simulink model "roach2_5gadc_spec"  (R2013b)
(part 3 of 18)

  pol1_in3_tap3/3(coeff_out) -> pol1_in3_tap4/3(coeff)
  pol1_in3_tap3/4(taps_out) -> adder_1_3/4(din3)
  pol1_in3_tap4/1(dout) -> pol1_in3_tap5/1(din)
  pol1_in3_tap4/2(sync_out) -> pol1_in3_tap5/2(sync)
  pol1_in3_tap4/3(coeff_out) -> pol1_in3_tap5/3(coeff)
  pol1_in3_tap4/4(taps_out) -> adder_1_3/5(din4)
  pol1_in3_tap5/1(dout) -> pol1_in3_tap6/1(din)
  pol1_in3_tap5/2(sync_out) -> pol1_in3_tap6/2(sync)
  pol1_in3_tap5/3(coeff_out) -> pol1_in3_tap6/3(coeff)
  pol1_in3_tap5/4(taps_out) -> adder_1_3/6(din5)
  pol1_in3_tap6/1(dout) -> pol1_in3_tap7/1(din)
  pol1_in3_tap6/2(sync_out) -> pol1_in3_tap7/2(sync)
  pol1_in3_tap6/3(coeff_out) -> pol1_in3_tap7/3(coeff)
  pol1_in3_tap6/4(taps_out) -> adder_1_3/7(din6)
  pol1_in3_last_tap/2(sync_out) -> adder_1_3/1(sync)
  pol1_in3_last_tap/1(tap_out) -> adder_1_3/9(din8)
  pol1_in3_tap7/1(dout) -> pol1_in3_last_tap/1(din)
  pol1_in3_tap7/2(sync_out) -> pol1_in3_last_tap/2(sync)
  pol1_in3_tap7/3(coeff_out) -> pol1_in3_last_tap/3(coeff)
  pol1_in3_tap7/4(taps_out) -> adder_1_3/8(din7)
  pol1_in4_first_tap/1(dout) -> pol1_in4_tap2/1(din)
  pol1_in4_first_tap/2(sync_out) -> pol1_in4_tap2/2(sync)
  pol1_in4_first_tap/3(coeff_out) -> pol1_in4_tap2/3(coeff)
  pol1_in4_first_tap/4(taps_out) -> adder_1_4/2(din1)
  pol1_in4_tap2/1(dout) -> pol1_in4_tap3/1(din)
  pol1_in4_tap2/2(sync_out) -> pol1_in4_tap3/2(sync)
  pol1_in4_tap2/3(coeff_out) -> pol1_in4_tap3/3(coeff)
  pol1_in4_tap2/4(taps_out) -> adder_1_4/3(din2)
  pol1_in4_tap3/1(dout) -> pol1_in4_tap4/1(din)
  pol1_in4_tap3/2(sync_out) -> pol1_in4_tap4/2(sync)
  pol1_in4_tap3/3(coeff_out) -> pol1_in4_tap4/3(coeff)
  pol1_in4_tap3/4(taps_out) -> adder_1_4/4(din3)
  pol1_in4_tap4/1(dout) -> pol1_in4_tap5/1(din)
  pol1_in4_tap4/2(sync_out) -> pol1_in4_tap5/2(sync)
  pol1_in4_tap4/3(coeff_out) -> pol1_in4_tap5/3(coeff)
  pol1_in4_tap4/4(taps_out) -> adder_1_4/5(din4)
  pol1_in4_tap5/1(dout) -> pol1_in4_tap6/1(din)
  pol1_in4_tap5/2(sync_out) -> pol1_in4_tap6/2(sync)
  pol1_in4_tap5/3(coeff_out) -> pol1_in4_tap6/3(coeff)
  pol1_in4_tap5/4(taps_out) -> adder_1_4/6(din5)
  pol1_in4_tap6/1(dout) -> pol1_in4_tap7/1(din)
  pol1_in4_tap6/2(sync_out) -> pol1_in4_tap7/2(sync)
  pol1_in4_tap6/3(coeff_out) -> pol1_in4_tap7/3(coeff)
  pol1_in4_tap6/4(taps_out) -> adder_1_4/7(din6)
  pol1_in4_last_tap/2(sync_out) -> adder_1_4/1(sync)
  pol1_in4_last_tap/1(tap_out) -> adder_1_4/9(din8)
  pol1_in4_tap7/1(dout) -> pol1_in4_last_tap/1(din)
  pol1_in4_tap7/2(sync_out) -> pol1_in4_last_tap/2(sync)
  pol1_in4_tap7/3(coeff_out) -> pol1_in4_last_tap/3(coeff)
  pol1_in4_tap7/4(taps_out) -> adder_1_4/8(din7)
  pol1_in5_first_tap/1(dout) -> pol1_in5_tap2/1(din)
  pol1_in5_first_tap/2(sync_out) -> pol1_in5_tap2/2(sync)
  pol1_in5_first_tap/3(coeff_out) -> pol1_in5_tap2/3(coeff)
  pol1_in5_first_tap/4(taps_out) -> adder_1_5/2(din1)
  pol1_in5_tap2/1(dout) -> pol1_in5_tap3/1(din)
  pol1_in5_tap2/2(sync_out) -> pol1_in5_tap3/2(sync)
  pol1_in5_tap2/3(coeff_out) -> pol1_in5_tap3/3(coeff)
  pol1_in5_tap2/4(taps_out) -> adder_1_5/3(din2)
  pol1_in5_tap3/1(dout) -> pol1_in5_tap4/1(din)
  pol1_in5_tap3/2(sync_out) -> pol1_in5_tap4/2(sync)
  pol1_in5_tap3/3(coeff_out) -> pol1_in5_tap4/3(coeff)
  pol1_in5_tap3/4(taps_out) -> adder_1_5/4(din3)
  pol1_in5_tap4/1(dout) -> pol1_in5_tap5/1(din)
  pol1_in5_tap4/2(sync_out) -> pol1_in5_tap5/2(sync)
  pol1_in5_tap4/3(coeff_out) -> pol1_in5_tap5/3(coeff)
  pol1_in5_tap4/4(taps_out) -> adder_1_5/5(din4)
  pol1_in5_tap5/1(dout) -> pol1_in5_tap6/1(din)
  pol1_in5_tap5/2(sync_out) -> pol1_in5_tap6/2(sync)
  pol1_in5_tap5/3(coeff_out) -> pol1_in5_tap6/3(coeff)
  pol1_in5_tap5/4(taps_out) -> adder_1_5/6(din5)
  pol1_in5_tap6/1(dout) -> pol1_in5_tap7/1(din)
  pol1_in5_tap6/2(sync_out) -> pol1_in5_tap7/2(sync)
  pol1_in5_tap6/3(coeff_out) -> pol1_in5_tap7/3(coeff)
  pol1_in5_tap6/4(taps_out) -> adder_1_5/7(din6)
  pol1_in5_last_tap/2(sync_out) -> adder_1_5/1(sync)
  pol1_in5_last_tap/1(tap_out) -> adder_1_5/9(din8)
  pol1_in5_tap7/1(dout) -> pol1_in5_last_tap/1(din)
  pol1_in5_tap7/2(sync_out) -> pol1_in5_last_tap/2(sync)
  pol1_in5_tap7/3(coeff_out) -> pol1_in5_last_tap/3(coeff)
  pol1_in5_tap7/4(taps_out) -> adder_1_5/8(din7)
  pol1_in6_first_tap/1(dout) -> pol1_in6_tap2/1(din)
  pol1_in6_first_tap/2(sync_out) -> pol1_in6_tap2/2(sync)
  pol1_in6_first_tap/3(coeff_out) -> pol1_in6_tap2/3(coeff)
  pol1_in6_first_tap/4(taps_out) -> adder_1_6/2(din1)
  pol1_in6_tap2/1(dout) -> pol1_in6_tap3/1(din)
  pol1_in6_tap2/2(sync_out) -> pol1_in6_tap3/2(sync)
  pol1_in6_tap2/3(coeff_out) -> pol1_in6_tap3/3(coeff)
  pol1_in6_tap2/4(taps_out) -> adder_1_6/3(din2)
  pol1_in6_tap3/1(dout) -> pol1_in6_tap4/1(din)
  pol1_in6_tap3/2(sync_out) -> pol1_in6_tap4/2(sync)
  pol1_in6_tap3/3(coeff_out) -> pol1_in6_tap4/3(coeff)
  pol1_in6_tap3/4(taps_out) -> adder_1_6/4(din3)
  pol1_in6_tap4/1(dout) -> pol1_in6_tap5/1(din)
  pol1_in6_tap4/2(sync_out) -> pol1_in6_tap5/2(sync)
  pol1_in6_tap4/3(coeff_out) -> pol1_in6_tap5/3(coeff)
  pol1_in6_tap4/4(taps_out) -> adder_1_6/5(din4)
  pol1_in6_tap5/1(dout) -> pol1_in6_tap6/1(din)
  pol1_in6_tap5/2(sync_out) -> pol1_in6_tap6/2(sync)
  pol1_in6_tap5/3(coeff_out) -> pol1_in6_tap6/3(coeff)
  pol1_in6_tap5/4(taps_out) -> adder_1_6/6(din5)
  pol1_in6_tap6/1(dout) -> pol1_in6_tap7/1(din)
  pol1_in6_tap6/2(sync_out) -> pol1_in6_tap7/2(sync)
  pol1_in6_tap6/3(coeff_out) -> pol1_in6_tap7/3(coeff)
  pol1_in6_tap6/4(taps_out) -> adder_1_6/7(din6)
  pol1_in6_last_tap/2(sync_out) -> adder_1_6/1(sync)
  pol1_in6_last_tap/1(tap_out) -> adder_1_6/9(din8)
  pol1_in6_tap7/1(dout) -> pol1_in6_last_tap/1(din)
  pol1_in6_tap7/2(sync_out) -> pol1_in6_last_tap/2(sync)
  pol1_in6_tap7/3(coeff_out) -> pol1_in6_last_tap/3(coeff)
  pol1_in6_tap7/4(taps_out) -> adder_1_6/8(din7)
  pol1_in7_first_tap/1(dout) -> pol1_in7_tap2/1(din)
  pol1_in7_first_tap/2(sync_out) -> pol1_in7_tap2/2(sync)
  pol1_in7_first_tap/3(coeff_out) -> pol1_in7_tap2/3(coeff)
  pol1_in7_first_tap/4(taps_out) -> adder_1_7/2(din1)
  pol1_in7_tap2/1(dout) -> pol1_in7_tap3/1(din)
  pol1_in7_tap2/2(sync_out) -> pol1_in7_tap3/2(sync)
  pol1_in7_tap2/3(coeff_out) -> pol1_in7_tap3/3(coeff)
  pol1_in7_tap2/4(taps_out) -> adder_1_7/3(din2)
  pol1_in7_tap3/1(dout) -> pol1_in7_tap4/1(din)
  pol1_in7_tap3/2(sync_out) -> pol1_in7_tap4/2(sync)
  pol1_in7_tap3/3(coeff_out) -> pol1_in7_tap4/3(coeff)
  pol1_in7_tap3/4(taps_out) -> adder_1_7/4(din3)
  pol1_in7_tap4/1(dout) -> pol1_in7_tap5/1(din)
  pol1_in7_tap4/2(sync_out) -> pol1_in7_tap5/2(sync)
  pol1_in7_tap4/3(coeff_out) -> pol1_in7_tap5/3(coeff)
  pol1_in7_tap4/4(taps_out) -> adder_1_7/5(din4)
  pol1_in7_tap5/1(dout) -> pol1_in7_tap6/1(din)
  pol1_in7_tap5/2(sync_out) -> pol1_in7_tap6/2(sync)
  pol1_in7_tap5/3(coeff_out) -> pol1_in7_tap6/3(coeff)
  pol1_in7_tap5/4(taps_out) -> adder_1_7/6(din5)
  pol1_in7_tap6/1(dout) -> pol1_in7_tap7/1(din)
  pol1_in7_tap6/2(sync_out) -> pol1_in7_tap7/2(sync)
  pol1_in7_tap6/3(coeff_out) -> pol1_in7_tap7/3(coeff)
  pol1_in7_tap6/4(taps_out) -> adder_1_7/7(din6)
  pol1_in7_last_tap/2(sync_out) -> adder_1_7/1(sync)
  pol1_in7_last_tap/1(tap_out) -> adder_1_7/9(din8)
  pol1_in7_tap7/1(dout) -> pol1_in7_last_tap/1(din)
  pol1_in7_tap7/2(sync_out) -> pol1_in7_last_tap/2(sync)
  pol1_in7_tap7/3(coeff_out) -> pol1_in7_last_tap/3(coeff)
  pol1_in7_tap7/4(taps_out) -> adder_1_7/8(din7)
  pol1_in8_first_tap/1(dout) -> pol1_in8_tap2/1(din)
  pol1_in8_first_tap/2(sync_out) -> pol1_in8_tap2/2(sync)
  pol1_in8_first_tap/3(coeff_out) -> pol1_in8_tap2/3(coeff)
  pol1_in8_first_tap/4(taps_out) -> adder_1_8/2(din1)
  pol1_in8_tap2/1(dout) -> pol1_in8_tap3/1(din)
  pol1_in8_tap2/2(sync_out) -> pol1_in8_tap3/2(sync)
  pol1_in8_tap2/3(coeff_out) -> pol1_in8_tap3/3(coeff)
  pol1_in8_tap2/4(taps_out) -> adder_1_8/3(din2)
  pol1_in8_tap3/1(dout) -> pol1_in8_tap4/1(din)
  pol1_in8_tap3/2(sync_out) -> pol1_in8_tap4/2(sync)
  pol1_in8_tap3/3(coeff_out) -> pol1_in8_tap4/3(coeff)
  pol1_in8_tap3/4(taps_out) -> adder_1_8/4(din3)
  pol1_in8_tap4/1(dout) -> pol1_in8_tap5/1(din)
  pol1_in8_tap4/2(sync_out) -> pol1_in8_tap5/2(sync)
  pol1_in8_tap4/3(coeff_out) -> pol1_in8_tap5/3(coeff)
  pol1_in8_tap4/4(taps_out) -> adder_1_8/5(din4)
  pol1_in8_tap5/1(dout) -> pol1_in8_tap6/1(din)
  pol1_in8_tap5/2(sync_out) -> pol1_in8_tap6/2(sync)
  pol1_in8_tap5/3(coeff_out) -> pol1_in8_tap6/3(coeff)
  pol1_in8_tap5/4(taps_out) -> adder_1_8/6(din5)
  pol1_in8_tap6/1(dout) -> pol1_in8_tap7/1(din)
  pol1_in8_tap6/2(sync_out) -> pol1_in8_tap7/2(sync)
  pol1_in8_tap6/3(coeff_out) -> pol1_in8_tap7/3(coeff)
  pol1_in8_tap6/4(taps_out) -> adder_1_8/7(din6)
  pol1_in8_last_tap/2(sync_out) -> adder_1_8/1(sync)
  pol1_in8_last_tap/1(tap_out) -> adder_1_8/9(din8)
  pol1_in8_tap7/1(dout) -> pol1_in8_last_tap/1(din)
  pol1_in8_tap7/2(sync_out) -> pol1_in8_last_tap/2(sync)
  pol1_in8_tap7/3(coeff_out) -> pol1_in8_last_tap/3(coeff)
  pol1_in8_tap7/4(taps_out) -> adder_1_8/8(din7)
  pol1_in9_first_tap/1(dout) -> pol1_in9_tap2/1(din)
  pol1_in9_first_tap/2(sync_out) -> pol1_in9_tap2/2(sync)
  pol1_in9_first_tap/3(coeff_out) -> pol1_in9_tap2/3(coeff)
  pol1_in9_first_tap/4(taps_out) -> adder_1_9/2(din1)
  pol1_in9_tap2/1(dout) -> pol1_in9_tap3/1(din)
  pol1_in9_tap2/2(sync_out) -> pol1_in9_tap3/2(sync)
  pol1_in9_tap2/3(coeff_out) -> pol1_in9_tap3/3(coeff)
  pol1_in9_tap2/4(taps_out) -> adder_1_9/3(din2)
  pol1_in9_tap3/1(dout) -> pol1_in9_tap4/1(din)
  pol1_in9_tap3/2(sync_out) -> pol1_in9_tap4/2(sync)
  pol1_in9_tap3/3(coeff_out) -> pol1_in9_tap4/3(coeff)
  pol1_in9_tap3/4(taps_out) -> adder_1_9/4(din3)
  pol1_in9_tap4/1(dout) -> pol1_in9_tap5/1(din)
  pol1_in9_tap4/2(sync_out) -> pol1_in9_tap5/2(sync)
  pol1_in9_tap4/3(coeff_out) -> pol1_in9_tap5/3(coeff)
  pol1_in9_tap4/4(taps_out) -> adder_1_9/5(din4)
  pol1_in9_tap5/1(dout) -> pol1_in9_tap6/1(din)
  pol1_in9_tap5/2(sync_out) -> pol1_in9_tap6/2(sync)
  pol1_in9_tap5/3(coeff_out) -> pol1_in9_tap6/3(coeff)
  pol1_in9_tap5/4(taps_out) -> adder_1_9/6(din5)
  pol1_in9_tap6/1(dout) -> pol1_in9_tap7/1(din)
  pol1_in9_tap6/2(sync_out) -> pol1_in9_tap7/2(sync)
  pol1_in9_tap6/3(coeff_out) -> pol1_in9_tap7/3(coeff)
  pol1_in9_tap6/4(taps_out) -> adder_1_9/7(din6)
  pol1_in9_last_tap/2(sync_out) -> adder_1_9/1(sync)
  pol1_in9_last_tap/1(tap_out) -> adder_1_9/9(din8)
  pol1_in9_tap7/1(dout) -> pol1_in9_last_tap/1(din)
  pol1_in9_tap7/2(sync_out) -> pol1_in9_last_tap/2(sync)
  pol1_in9_tap7/3(coeff_out) -> pol1_in9_last_tap/3(coeff)
  pol1_in9_tap7/4(taps_out) -> adder_1_9/8(din7)
  pol1_in10_first_tap/1(dout) -> pol1_in10_tap2/1(din)
  pol1_in10_first_tap/2(sync_out) -> pol1_in10_tap2/2(sync)
  pol1_in10_first_tap/3(coeff_out) -> pol1_in10_tap2/3(coeff)
  pol1_in10_first_tap/4(taps_out) -> adder_1_10/2(din1)
  pol1_in10_tap2/1(dout) -> pol1_in10_tap3/1(din)
  pol1_in10_tap2/2(sync_out) -> pol1_in10_tap3/2(sync)
  pol1_in10_tap2/3(coeff_out) -> pol1_in10_tap3/3(coeff)
  pol1_in10_tap2/4(taps_out) -> adder_1_10/3(din2)
  pol1_in10_tap3/1(dout) -> pol1_in10_tap4/1(din)
  pol1_in10_tap3/2(sync_out) -> pol1_in10_tap4/2(sync)
  pol1_in10_tap3/3(coeff_out) -> pol1_in10_tap4/3(coeff)
  pol1_in10_tap3/4(taps_out) -> adder_1_10/4(din3)
  pol1_in10_tap4/1(dout) -> pol1_in10_tap5/1(din)
  pol1_in10_tap4/2(sync_out) -> pol1_in10_tap5/2(sync)
  pol1_in10_tap4/3(coeff_out) -> pol1_in10_tap5/3(coeff)
  pol1_in10_tap4/4(taps_out) -> adder_1_10/5(din4)
  pol1_in10_tap5/1(dout) -> pol1_in10_tap6/1(din)
  pol1_in10_tap5/2(sync_out) -> pol1_in10_tap6/2(sync)
  pol1_in10_tap5/3(coeff_out) -> pol1_in10_tap6/3(coeff)
  pol1_in10_tap5/4(taps_out) -> adder_1_10/6(din5)
  pol1_in10_tap6/1(dout) -> pol1_in10_tap7/1(din)
  pol1_in10_tap6/2(sync_out) -> pol1_in10_tap7/2(sync)
  pol1_in10_tap6/3(coeff_out) -> pol1_in10_tap7/3(coeff)
  pol1_in10_tap6/4(taps_out) -> adder_1_10/7(din6)
  pol1_in10_last_tap/2(sync_out) -> adder_1_10/1(sync)
  pol1_in10_last_tap/1(tap_out) -> adder_1_10/9(din8)
  pol1_in10_tap7/1(dout) -> pol1_in10_last_tap/1(din)
  pol1_in10_tap7/2(sync_out) -> pol1_in10_last_tap/2(sync)
  pol1_in10_tap7/3(coeff_out) -> pol1_in10_last_tap/3(coeff)
  pol1_in10_tap7/4(taps_out) -> adder_1_10/8(din7)
  pol1_in11_first_tap/1(dout) -> pol1_in11_tap2/1(din)
  pol1_in11_first_tap/2(sync_out) -> pol1_in11_tap2/2(sync)
  pol1_in11_first_tap/3(coeff_out) -> pol1_in11_tap2/3(coeff)
  pol1_in11_first_tap/4(taps_out) -> adder_1_11/2(din1)
  pol1_in11_tap2/1(dout) -> pol1_in11_tap3/1(din)
  pol1_in11_tap2/2(sync_out) -> pol1_in11_tap3/2(sync)
  pol1_in11_tap2/3(coeff_out) -> pol1_in11_tap3/3(coeff)
  pol1_in11_tap2/4(taps_out) -> adder_1_11/3(din2)
  pol1_in11_tap3/1(dout) -> pol1_in11_tap4/1(din)
  pol1_in11_tap3/2(sync_out) -> pol1_in11_tap4/2(sync)
  pol1_in11_tap3/3(coeff_out) -> pol1_in11_tap4/3(coeff)
  pol1_in11_tap3/4(taps_out) -> adder_1_11/4(din3)
  pol1_in11_tap4/1(dout) -> pol1_in11_tap5/1(din)
  pol1_in11_tap4/2(sync_out) -> pol1_in11_tap5/2(sync)
  pol1_in11_tap4/3(coeff_out) -> pol1_in11_tap5/3(coeff)
  pol1_in11_tap4/4(taps_out) -> adder_1_11/5(din4)
  pol1_in11_tap5/1(dout) -> pol1_in11_tap6/1(din)
  pol1_in11_tap5/2(sync_out) -> pol1_in11_tap6/2(sync)
  pol1_in11_tap5/3(coeff_out) -> pol1_in11_tap6/3(coeff)
  pol1_in11_tap5/4(taps_out) -> adder_1_11/6(din5)
  pol1_in11_tap6/1(dout) -> pol1_in11_tap7/1(din)
  pol1_in11_tap6/2(sync_out) -> pol1_in11_tap7/2(sync)
  pol1_in11_tap6/3(coeff_out) -> pol1_in11_tap7/3(coeff)
  pol1_in11_tap6/4(taps_out) -> adder_1_11/7(din6)
  pol1_in11_last_tap/2(sync_out) -> adder_1_11/1(sync)
  pol1_in11_last_tap/1(tap_out) -> adder_1_11/9(din8)
  pol1_in11_tap7/1(dout) -> pol1_in11_last_tap/1(din)
  pol1_in11_tap7/2(sync_out) -> pol1_in11_last_tap/2(sync)
  pol1_in11_tap7/3(coeff_out) -> pol1_in11_last_tap/3(coeff)
  pol1_in11_tap7/4(taps_out) -> adder_1_11/8(din7)
  pol1_in12_first_tap/1(dout) -> pol1_in12_tap2/1(din)
  pol1_in12_first_tap/2(sync_out) -> pol1_in12_tap2/2(sync)
  pol1_in12_first_tap/3(coeff_out) -> pol1_in12_tap2/3(coeff)
  pol1_in12_first_tap/4(taps_out) -> adder_1_12/2(din1)
  pol1_in12_tap2/1(dout) -> pol1_in12_tap3/1(din)
  pol1_in12_tap2/2(sync_out) -> pol1_in12_tap3/2(sync)
  pol1_in12_tap2/3(coeff_out) -> pol1_in12_tap3/3(coeff)
  pol1_in12_tap2/4(taps_out) -> adder_1_12/3(din2)
  pol1_in12_tap3/1(dout) -> pol1_in12_tap4/1(din)
  pol1_in12_tap3/2(sync_out) -> pol1_in12_tap4/2(sync)
  pol1_in12_tap3/3(coeff_out) -> pol1_in12_tap4/3(coeff)
  pol1_in12_tap3/4(taps_out) -> adder_1_12/4(din3)
  pol1_in12_tap4/1(dout) -> pol1_in12_tap5/1(din)
  pol1_in12_tap4/2(sync_out) -> pol1_in12_tap5/2(sync)
  pol1_in12_tap4/3(coeff_out) -> pol1_in12_tap5/3(coeff)
  pol1_in12_tap4/4(taps_out) -> adder_1_12/5(din4)
  pol1_in12_tap5/1(dout) -> pol1_in12_tap6/1(din)
  pol1_in12_tap5/2(sync_out) -> pol1_in12_tap6/2(sync)
  pol1_in12_tap5/3(coeff_out) -> pol1_in12_tap6/3(coeff)
  pol1_in12_tap5/4(taps_out) -> adder_1_12/6(din5)
  pol1_in12_tap6/1(dout) -> pol1_in12_tap7/1(din)
  pol1_in12_tap6/2(sync_out) -> pol1_in12_tap7/2(sync)
  pol1_in12_tap6/3(coeff_out) -> pol1_in12_tap7/3(coeff)
  pol1_in12_tap6/4(taps_out) -> adder_1_12/7(din6)
  pol1_in12_last_tap/2(sync_out) -> adder_1_12/1(sync)
  pol1_in12_last_tap/1(tap_out) -> adder_1_12/9(din8)
  pol1_in12_tap7/1(dout) -> pol1_in12_last_tap/1(din)
  pol1_in12_tap7/2(sync_out) -> pol1_in12_last_tap/2(sync)
  pol1_in12_tap7/3(coeff_out) -> pol1_in12_last_tap/3(coeff)
  pol1_in12_tap7/4(taps_out) -> adder_1_12/8(din7)
  pol1_in13_first_tap/1(dout) -> pol1_in13_tap2/1(din)
  pol1_in13_first_tap/2(sync_out) -> pol1_in13_tap2/2(sync)
  pol1_in13_first_tap/3(coeff_out) -> pol1_in13_tap2/3(coeff)
  pol1_in13_first_tap/4(taps_out) -> adder_1_13/2(din1)
  pol1_in13_tap2/1(dout) -> pol1_in13_tap3/1(din)
  pol1_in13_tap2/2(sync_out) -> pol1_in13_tap3/2(sync)
  pol1_in13_tap2/3(coeff_out) -> pol1_in13_tap3/3(coeff)
  pol1_in13_tap2/4(taps_out) -> adder_1_13/3(din2)
  pol1_in13_tap3/1(dout) -> pol1_in13_tap4/1(din)
  pol1_in13_tap3/2(sync_out) -> pol1_in13_tap4/2(sync)
  pol1_in13_tap3/3(coeff_out) -> pol1_in13_tap4/3(coeff)
  pol1_in13_tap3/4(taps_out) -> adder_1_13/4(din3)
  pol1_in13_tap4/1(dout) -> pol1_in13_tap5/1(din)
  pol1_in13_tap4/2(sync_out) -> pol1_in13_tap5/2(sync)
  pol1_in13_tap4/3(coeff_out) -> pol1_in13_tap5/3(coeff)
  pol1_in13_tap4/4(taps_out) -> adder_1_13/5(din4)
  pol1_in13_tap5/1(dout) -> pol1_in13_tap6/1(din)
  pol1_in13_tap5/2(sync_out) -> pol1_in13_tap6/2(sync)
  pol1_in13_tap5/3(coeff_out) -> pol1_in13_tap6/3(coeff)
  pol1_in13_tap5/4(taps_out) -> adder_1_13/6(din5)
  pol1_in13_tap6/1(dout) -> pol1_in13_tap7/1(din)
  pol1_in13_tap6/2(sync_out) -> pol1_in13_tap7/2(sync)
  pol1_in13_tap6/3(coeff_out) -> pol1_in13_tap7/3(coeff)
  pol1_in13_tap6/4(taps_out) -> adder_1_13/7(din6)
  pol1_in13_last_tap/2(sync_out) -> adder_1_13/1(sync)
  pol1_in13_last_tap/1(tap_out) -> adder_1_13/9(din8)
  pol1_in13_tap7/1(dout) -> pol1_in13_last_tap/1(din)
  pol1_in13_tap7/2(sync_out) -> pol1_in13_last_tap/2(sync)
  pol1_in13_tap7/3(coeff_out) -> pol1_in13_last_tap/3(coeff)
  pol1_in13_tap7/4(taps_out) -> adder_1_13/8(din7)
  pol1_in14_first_tap/1(dout) -> pol1_in14_tap2/1(din)
  pol1_in14_first_tap/2(sync_out) -> pol1_in14_tap2/2(sync)
  pol1_in14_first_tap/3(coeff_out) -> pol1_in14_tap2/3(coeff)
  pol1_in14_first_tap/4(taps_out) -> adder_1_14/2(din1)
  pol1_in14_tap2/1(dout) -> pol1_in14_tap3/1(din)
  pol1_in14_tap2/2(sync_out) -> pol1_in14_tap3/2(sync)
  pol1_in14_tap2/3(coeff_out) -> pol1_in14_tap3/3(coeff)
  pol1_in14_tap2/4(taps_out) -> adder_1_14/3(din2)
  pol1_in14_tap3/1(dout) -> pol1_in14_tap4/1(din)
  pol1_in14_tap3/2(sync_out) -> pol1_in14_tap4/2(sync)
  pol1_in14_tap3/3(coeff_out) -> pol1_in14_tap4/3(coeff)
  pol1_in14_tap3/4(taps_out) -> adder_1_14/4(din3)
  pol1_in14_tap4/1(dout) -> pol1_in14_tap5/1(din)
  pol1_in14_tap4/2(sync_out) -> pol1_in14_tap5/2(sync)
  pol1_in14_tap4/3(coeff_out) -> pol1_in14_tap5/3(coeff)
  pol1_in14_tap4/4(taps_out) -> adder_1_14/5(din4)
  pol1_in14_tap5/1(dout) -> pol1_in14_tap6/1(din)
  pol1_in14_tap5/2(sync_out) -> pol1_in14_tap6/2(sync)
  pol1_in14_tap5/3(coeff_out) -> pol1_in14_tap6/3(coeff)
  pol1_in14_tap5/4(taps_out) -> adder_1_14/6(din5)
  pol1_in14_tap6/1(dout) -> pol1_in14_tap7/1(din)
  pol1_in14_tap6/2(sync_out) -> pol1_in14_tap7/2(sync)
  pol1_in14_tap6/3(coeff_out) -> pol1_in14_tap7/3(coeff)
  pol1_in14_tap6/4(taps_out) -> adder_1_14/7(din6)
  pol1_in14_last_tap/2(sync_out) -> adder_1_14/1(sync)
  pol1_in14_last_tap/1(tap_out) -> adder_1_14/9(din8)
  pol1_in14_tap7/1(dout) -> pol1_in14_last_tap/1(din)
  pol1_in14_tap7/2(sync_out) -> pol1_in14_last_tap/2(sync)
  pol1_in14_tap7/3(coeff_out) -> pol1_in14_last_tap/3(coeff)
  pol1_in14_tap7/4(taps_out) -> adder_1_14/8(din7)
  pol1_in15_first_tap/1(dout) -> pol1_in15_tap2/1(din)
  pol1_in15_first_tap/2(sync_out) -> pol1_in15_tap2/2(sync)
  pol1_in15_first_tap/3(coeff_out) -> pol1_in15_tap2/3(coeff)
  pol1_in15_first_tap/4(taps_out) -> adder_1_15/2(din1)
  pol1_in15_tap2/1(dout) -> pol1_in15_tap3/1(din)
  pol1_in15_tap2/2(sync_out) -> pol1_in15_tap3/2(sync)
  pol1_in15_tap2/3(coeff_out) -> pol1_in15_tap3/3(coeff)
  pol1_in15_tap2/4(taps_out) -> adder_1_15/3(din2)
  pol1_in15_tap3/1(dout) -> pol1_in15_tap4/1(din)
  pol1_in15_tap3/2(sync_out) -> pol1_in15_tap4/2(sync)
  pol1_in15_tap3/3(coeff_out) -> pol1_in15_tap4/3(coeff)
  pol1_in15_tap3/4(taps_out) -> adder_1_15/4(din3)
  pol1_in15_tap4/1(dout) -> pol1_in15_tap5/1(din)
  pol1_in15_tap4/2(sync_out) -> pol1_in15_tap5/2(sync)
  pol1_in15_tap4/3(coeff_out) -> pol1_in15_tap5/3(coeff)
  pol1_in15_tap4/4(taps_out) -> adder_1_15/5(din4)
  pol1_in15_tap5/1(dout) -> pol1_in15_tap6/1(din)
  pol1_in15_tap5/2(sync_out) -> pol1_in15_tap6/2(sync)
  pol1_in15_tap5/3(coeff_out) -> pol1_in15_tap6/3(coeff)
  pol1_in15_tap5/4(taps_out) -> adder_1_15/6(din5)
  pol1_in15_tap6/1(dout) -> pol1_in15_tap7/1(din)
  pol1_in15_tap6/2(sync_out) -> pol1_in15_tap7/2(sync)
  pol1_in15_tap6/3(coeff_out) -> pol1_in15_tap7/3(coeff)
  pol1_in15_tap6/4(taps_out) -> adder_1_15/7(din6)
  pol1_in15_last_tap/2(sync_out) -> adder_1_15/1(sync)
  pol1_in15_last_tap/1(tap_out) -> adder_1_15/9(din8)
  pol1_in15_tap7/1(dout) -> pol1_in15_last_tap/1(din)
  pol1_in15_tap7/2(sync_out) -> pol1_in15_last_tap/2(sync)
  pol1_in15_tap7/3(coeff_out) -> pol1_in15_last_tap/3(coeff)
  pol1_in15_tap7/4(taps_out) -> adder_1_15/8(din7)
  pol1_in16_first_tap/1(dout) -> pol1_in16_tap2/1(din)
  pol1_in16_first_tap/2(sync_out) -> pol1_in16_tap2/2(sync)
  pol1_in16_first_tap/3(coeff_out) -> pol1_in16_tap2/3(coeff)
  pol1_in16_first_tap/4(taps_out) -> adder_1_16/2(din1)
  pol1_in16_tap2/1(dout) -> pol1_in16_tap3/1(din)
  pol1_in16_tap2/2(sync_out) -> pol1_in16_tap3/2(sync)
  pol1_in16_tap2/3(coeff_out) -> pol1_in16_tap3/3(coeff)
  pol1_in16_tap2/4(taps_out) -> adder_1_16/3(din2)
  pol1_in16_tap3/1(dout) -> pol1_in16_tap4/1(din)
  pol1_in16_tap3/2(sync_out) -> pol1_in16_tap4/2(sync)
  pol1_in16_tap3/3(coeff_out) -> pol1_in16_tap4/3(coeff)
  pol1_in16_tap3/4(taps_out) -> adder_1_16/4(din3)
  pol1_in16_tap4/1(dout) -> pol1_in16_tap5/1(din)
  pol1_in16_tap4/2(sync_out) -> pol1_in16_tap5/2(sync)
  pol1_in16_tap4/3(coeff_out) -> pol1_in16_tap5/3(coeff)
  pol1_in16_tap4/4(taps_out) -> adder_1_16/5(din4)
  pol1_in16_tap5/1(dout) -> pol1_in16_tap6/1(din)
  pol1_in16_tap5/2(sync_out) -> pol1_in16_tap6/2(sync)
  pol1_in16_tap5/3(coeff_out) -> pol1_in16_tap6/3(coeff)
  pol1_in16_tap5/4(taps_out) -> adder_1_16/6(din5)
  pol1_in16_tap6/1(dout) -> pol1_in16_tap7/1(din)
  pol1_in16_tap6/2(sync_out) -> pol1_in16_tap7/2(sync)
  pol1_in16_tap6/3(coeff_out) -> pol1_in16_tap7/3(coeff)
  pol1_in16_tap6/4(taps_out) -> adder_1_16/7(din6)
  pol1_in16_last_tap/2(sync_out) -> adder_1_16/1(sync)
  pol1_in16_last_tap/1(tap_out) -> adder_1_16/9(din8)
  pol1_in16_tap7/1(dout) -> pol1_in16_last_tap/1(din)
  pol1_in16_tap7/2(sync_out) -> pol1_in16_last_tap/2(sync)
  pol1_in16_tap7/3(coeff_out) -> pol1_in16_last_tap/3(coeff)
  pol1_in16_tap7/4(taps_out) -> adder_1_16/8(din7)
